simulink library "casper_library_sources"  (Simulink 7.0)
values from neighbouring files (symbols this model uses):
  quant = 'Round  (unbiased: +/- Inf)'    [bus_add_init.m]    (also in bus_addsub_init.m; bus_convert_init.m = 'Round  (unbiased: Even Values)'; bus_maddsub_init.m; bus_mult_init.m)
libraries: xbsIndex_r4 x42, casper_library_sources x2
settings Model: Creator=mdexter  LastModifiedBy=mdexter

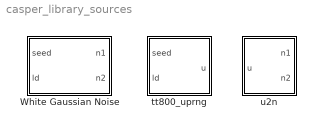
== system casper_library_sources ==
  White Gaussian Noise : Subsystem  mask(White Gaussian Noise Generator){seed=hex2dec('12345678')}
      mask help: Outputs two independent white gaussian noise signals as Fix_17_14 values with standard deviation 1.0, expected value 0.0, and crest factor 3.90625 (125/32).
      mask Help:
      | Initial seed is specified by a mask parameter at design time.  Can be reseeded at runtime by applying a UFix_32_0 value on the seed input and pulsing the load port (ld) high for one cycle.  Holding the load port high for more than one cycle is allowed, but it affects the underlying PRNG in undocumented ways.  Drill down into the subsystem if you want to learn more.
      | 
      | This block uses a TT800 uniform pseudo-random number generator followed by a uniform-to-normal converter implementing the Box-Muller Polar algorithm.
      | 
      | The TT800 is a high quality pseudo-random number generator based on a "twisted generialized linear feedback shift register".  Its output sequence repeats after 2^800 samples (~10^240 samples).  For more info see: Matsumoto, M. and Kurita, Y. 1994. "Twisted GFSR generators II", ACM Trans. Model. Comput. Simul. 4, 3 (Jul. 1994), 254-266 (http://doi.acm.org/10.1145/189443.189445).
      mask CallbackString:
      | if str2num(get_param(gcb, 'seed')) == 0
      |     error('Seed cannot be zero.')
      | end
      mask Display:
      | port_label('input',1,'seed');
      | port_label('input',2,'ld');
      | port_label('output',1,'n1');
      | port_label('output',2,'n2');
  tt800_uprng : Subsystem  mask(TT800 Uniform Psedo-Random Number Generator){seed=hex2dec('12345678')}
      mask help: The TT800 is a high quality pseudo-random number generator based on a "twisted generialized linear feedback shift register". Its output sequence repeats after 2^800 samples (~10^240 samples). For more info see: Matsumoto, M. and Kurita, Y. 1994. "Twisted GFSR generators II", ACM Trans. Model. Comput. Simul. 4, 3 (Jul. 1994), 254-266 (http://doi.acm.org/10.1145/189443.189445).
      mask init:
      | set_param([gcb,'/tt800_seed_gen/LFSR'],'rst_value',sprintf('''%08X''', seed));
      mask Help: Initial seed is specified by a mask parameter at design time.  Can be reseeded at runtime by applying a UFix_32_0 value on the seed input and pulsing the load port (ld) high for one cycle.  Holding the load port high for more than one cycle is allowed, but it affects the generator in undocumented ways.  Drill down into the subsystem if you want to learn more.
      mask Display:
      | port_label('input',1,'seed');
      | port_label('input',2,'ld');
      | port_label('output',1,'u');
  u2n : Subsystem  mask(Uniform to Normal Converter){hideme=off}
      mask prompts: hideme "Hide me"
      mask help: Converts a variable with uniform distribution into two independent normally distributed variables.
      mask Help: Converts a variable with uniform distribution into two independent normally distributed variables.

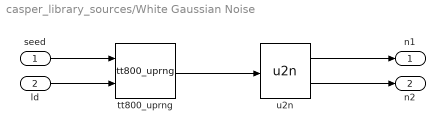
== system casper_library_sources/White Gaussian Noise ==
  seed : Inport  OutDataType=sfix(16)  OutScaling=2^0
  ld : Inport  Port=2  OutDataType=sfix(16)  OutScaling=2^0
  tt800_uprng : casper_library_sources/tt800_uprng  SystemSampleTime=-1  seed=seed
  u2n : casper_library_sources/u2n  SystemSampleTime=-1  hideme=off
  n1 : Outport  OutDataType=sfix(16)  OutScaling=2^0
  n2 : Outport  Port=2  OutDataType=sfix(16)  OutScaling=2^0
  wires:
  tt800_uprng/1 -> u2n/1
  seed/1 -> tt800_uprng/1
  u2n/1 -> n1/1
  ld/1 -> tt800_uprng/2
  u2n/2 -> n2/1

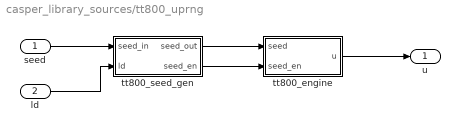
== system casper_library_sources/tt800_uprng ==
  seed : Inport  OutDataType=sfix(16)  OutScaling=2^0
  ld : Inport  Port=2  OutDataType=sfix(16)  OutScaling=2^0
  tt800_engine : Subsystem
  tt800_seed_gen : Subsystem
  u : Outport  OutDataType=sfix(16)  OutScaling=2^0
  wires:
  ld/1 -> tt800_seed_gen/2(ld)
  tt800_engine/1(u) -> u/1
  seed/1 -> tt800_seed_gen/1(seed_in)
  tt800_seed_gen/2(seed_en) -> tt800_engine/2(seed_en)
  tt800_seed_gen/1(seed_out) -> tt800_engine/1(seed)

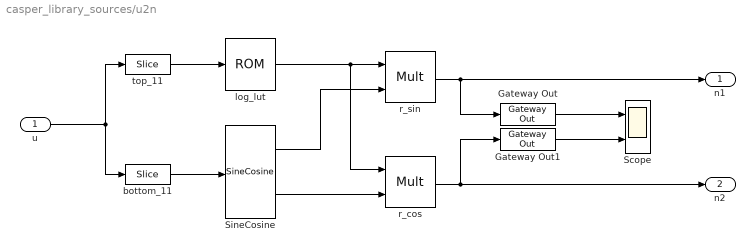
== system casper_library_sources/u2n ==
  u : Inport  OutDataType=sfix(16)  OutScaling=2^0
  Gateway Out : xbsIndex_r4/Gateway Out  hdl_port=off  timing_constraint=None  locs_specified=off  LOCs={}  block_type=gatewayout
      settings: infoedit="Gateway out block.  Converts Xilinx fixed point inputs into ouputs of type Simulink integer, double, or fixed point.<P><P>Hardware notes:  In hardware these blocks become top level output ports or are discarded, depending on how they are configured."  xl_area=[0 0 0 0 17 0 0]  block_version=10.1.3
  Gateway Out1 : xbsIndex_r4/Gateway Out  hdl_port=off  timing_constraint=None  locs_specified=off  LOCs={}  block_type=gatewayout
      settings: infoedit="Gateway out block.  Converts Xilinx fixed point inputs into ouputs of type Simulink integer, double, or fixed point.<P><P>Hardware notes:  In hardware these blocks become top level output ports or are discarded, depending on how they are configured."  xl_area=[0 0 0 0 17 0 0]  block_version=10.1.3
  Scope : Scope  NumInputPorts=2
      settings: YMin=-5~-5  YMax=5~5
  SineCosine : xbsIndex_r4/SineCosine  mode=Sine and Cosine  neg_sin=off  neg_cos=off  n_bits=8  sym_output=off  en=off  latency=2  dbl_ovrd=off  explicit_period=off  period=1  mem_type=Block RAM  pipeline=on  use_rpm=on  block_type=sincos
      settings: xl_area=[8 16 1 2 0 0 0]  block_version=10.1.3
  bottom_11 : xbsIndex_r4/Slice  nbits=11  boolean_output=off  mode=Lower Bit Location + Width  bit1=0  base1=MSB of Input  bit0=0  base0=LSB of Input  dbl_ovrd=off  block_type=slice
      settings: infoedit="Extracts a given range of bits from each input sample and presents it at the output.  The output type is ordinarily unsigned with binary point at zero, but can be Boolean when the slice is one bit wide.<P><P>Hardware notes: In hardware this block costs nothing."  block_version=10.1.3
  log_lut : xbsIndex_r4/ROM  depth=2^11  initVector=quant(sqrt(-2*log(linspace(2^-11,1,2^11))),2^-7)  distributed_mem=Block RAM  rst=off  init_reg=0  en=off  latency=1  arith_type=Unsigned  n_bits=9  bin_pt=7  dbl_ovrd=off  optimize=Area  use_rpm=off  block_type=sprom
      settings: xl_area=[0 0 1 0 0 0 0]  block_version=10.1.3
  r_cos : xbsIndex_r4/Mult  precision=Full  arith_type="Signed  (2's comp)"  n_bits=8  bin_pt=2  quantization=Truncate  overflow=Wrap  en=off  latency=3  dbl_ovrd=off  use_behavioral_HDL=off  use_embedded=on  opt=Speed  optimum_pipeline=off  pipeline=on  use_rpm=on  placement_style=Rectangular shape  block_type=mult
      settings: infoedit=Hardware notes: To use the internal pipeline stage of the dedicated multiplier you must select 'Pipeline for maximum performance'.  xl_area=[18 34 0 17 0 1 0]  block_version=10.1.3
  r_sin : xbsIndex_r4/Mult  precision=Full  arith_type="Signed  (2's comp)"  n_bits=8  bin_pt=2  quantization=Truncate  overflow=Wrap  en=off  latency=3  dbl_ovrd=off  use_behavioral_HDL=off  use_embedded=on  opt=Speed  optimum_pipeline=off  pipeline=on  use_rpm=on  placement_style=Rectangular shape  block_type=mult
      settings: infoedit=Hardware notes: To use the internal pipeline stage of the dedicated multiplier you must select 'Pipeline for maximum performance'.  xl_area=[18 34 0 17 0 1 0]  block_version=10.1.3
  top_11 : xbsIndex_r4/Slice  nbits=11  boolean_output=off  mode=Upper Bit Location + Width  bit1=0  base1=MSB of Input  bit0=0  base0=MSB of Input  dbl_ovrd=off  block_type=slice
      settings: infoedit="Extracts a given range of bits from each input sample and presents it at the output.  The output type is ordinarily unsigned with binary point at zero, but can be Boolean when the slice is one bit wide.<P><P>Hardware notes: In hardware this block costs nothing."  block_version=10.1.3
  n1 : Outport  OutDataType=sfix(16)  OutScaling=2^0
  n2 : Outport  Port=2  OutDataType=sfix(16)  OutScaling=2^0
  wires:
  r_cos/1 -> n2/1, Gateway Out1/1
  r_sin/1 -> n1/1, Gateway Out/1
  SineCosine/1 -> r_sin/2
  log_lut/1 -> r_cos/1, r_sin/1
  SineCosine/2 -> r_cos/2
  u/1 -> bottom_11/1, top_11/1
  top_11/1 -> log_lut/1
  bottom_11/1 -> SineCosine/1
  Gateway Out1/1 -> Scope/2
  Gateway Out/1 -> Scope/1

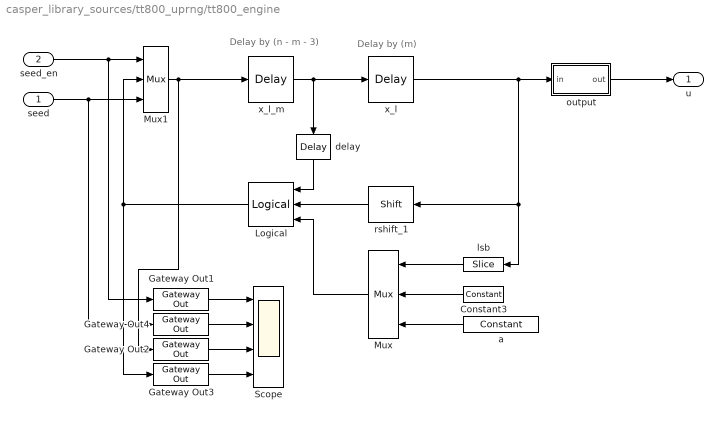
== system casper_library_sources/tt800_uprng/tt800_engine ==
  note: Delay by (m)
  note: Delay by (n - m - 3)
  seed : Inport  OutDataType=sfix(16)  OutScaling=2^0
  seed_en : Inport  Port=2  OutDataType=sfix(16)  OutScaling=2^0
  Constant3 : xbsIndex_r4/Constant  Orientation=left  arith_type=Unsigned  const=0  n_bits=32  bin_pt=0  explicit_period=off  period=1  equ=P=C  opselect=C  inp2=PCIN>>17  opr=+  inp1=P  carry=CIN  dbl_ovrd=off  block_type=constant
  Gateway Out{1..4} (4 alike) : xbsIndex_r4/Gateway Out  hdl_port=off  timing_constraint=None  locs_specified=off  LOCs={}  block_type=gatewayout
      settings: infoedit="Gateway out block.  Converts Xilinx fixed point inputs into ouputs of type Simulink integer, double, or fixed point.<P><P>Hardware notes:  In hardware these blocks become top level output ports or are discarded, depending on how they are configured."  xl_area=[0 0 0 0 0 0 0]  block_version=10.1.3
  Logical : xbsIndex_r4/Logical  Orientation=left  logical_function=XOR  inputs=3  en=off  latency=1  precision=Full  arith_type=Unsigned  n_bits=8  bin_pt=2  align_bp=off  dbl_ovrd=off  block_type=logical
      settings: xl_area=[32 32 0 32 0 0 0]
  Mux : xbsIndex_r4/Mux  Orientation=left  inputs=2  en=off  latency=1  precision=Full  arith_type="Signed  (2's comp)"  n_bits=8  bin_pt=2  quantization=Truncate  overflow=Wrap  dbl_ovrd=off  block_type=mux
      settings: xl_area=[16 32 0 32 0 0 0]
  Mux1 : xbsIndex_r4/Mux  inputs=2  en=off  latency=1  precision=Full  arith_type="Signed  (2's comp)"  n_bits=8  bin_pt=2  quantization=Truncate  overflow=Wrap  dbl_ovrd=off  block_type=mux
      settings: xl_area=[16 32 0 32 0 0 0]
  Scope : Scope  NumInputPorts=4
      settings: YMin=-5~-5~-5~-5  YMax=5~5~5~5
  a : xbsIndex_r4/Constant  Orientation=left  arith_type=Unsigned  const=hex2dec('8EBFD028')  n_bits=32  bin_pt=0  explicit_period=off  period=1  equ=P=C  opselect=C  inp2=PCIN>>17  opr=+  inp1=P  carry=CIN  dbl_ovrd=off  block_type=constant
  delay : xbsIndex_r4/Delay  Orientation=down  en=off  latency=1  dbl_ovrd=off  reg_retiming=off  block_type=delay
      settings: xl_area=[16 32 0 0 0 0 0]
  lsb : xbsIndex_r4/Slice  Orientation=left  nbits=1  boolean_output=off  mode=Lower Bit Location + Width  bit1=0  base1=MSB of Input  bit0=0  base0=LSB of Input  dbl_ovrd=off  block_type=slice
      settings: infoedit="Extracts a given range of bits from each input sample and presents it at the output.  The output type is ordinarily unsigned with binary point at zero, but can be Boolean when the slice is one bit wide.<P><P>Hardware notes: In hardware this block costs nothing."  block_version=10.1.3
  output : Subsystem
  rshift_1 : xbsIndex_r4/Shift  Orientation=left  shift_dir=Right  shift_bits=1  en=off  latency=1  precision=User Defined  arith_type=Unsigned  n_bits=32  bin_pt=0  quantization=Truncate  overflow=Wrap  dbl_ovrd=off  block_type=shift
      settings: xl_area=[0 32 0 0 0 0 0]  block_version=10.1.3
  x_l : xbsIndex_r4/Delay  en=off  latency=7  dbl_ovrd=off  reg_retiming=off  block_type=delay
      settings: xl_area=[16 32 0 32 0 0 0]
  x_l_m : xbsIndex_r4/Delay  en=off  latency=25-7-3  dbl_ovrd=off  reg_retiming=off  block_type=delay
      settings: xl_area=[16 32 0 32 0 0 0]
  u : Outport  OutDataType=sfix(16)  OutScaling=2^0
  wires:
  x_l_m/1 -> x_l/1, delay/1
  x_l/1 -> lsb/1, rshift_1/1, output/1(in)
  lsb/1 -> Mux/1
  Constant3/1 -> Mux/2
  a/1 -> Mux/3
  rshift_1/1 -> Logical/2
  Mux/1 -> Logical/3
  Logical/1 -> Gateway Out3/1, Mux1/2
  Mux1/1 -> x_l_m/1, Gateway Out2/1
  seed_en/1 -> Gateway Out1/1, Mux1/1
  seed/1 -> Gateway Out4/1, Mux1/3
  Gateway Out1/1 -> Scope/1
  Gateway Out4/1 -> Scope/2
  Gateway Out2/1 -> Scope/3
  Gateway Out3/1 -> Scope/4
  output/1(out) -> u/1
  delay/1 -> Logical/1

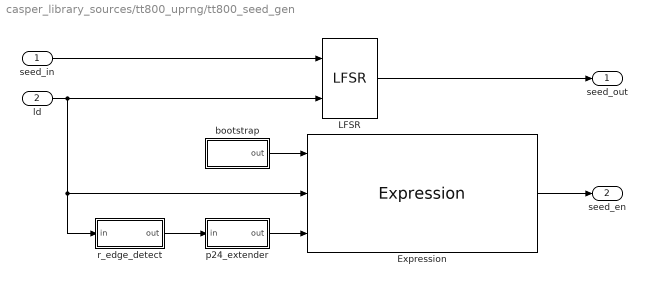
== system casper_library_sources/tt800_uprng/tt800_seed_gen ==
  seed_in : Inport  OutDataType=sfix(16)  OutScaling=2^0
  ld : Inport  Port=2  OutDataType=sfix(16)  OutScaling=2^0
  Expression : xbsIndex_r4/Expression  expression=(bootstrap | ld | ld_ext)  align_bp=on  en=off  latency=1  precision=Full  arith_type=Unsigned  n_bits=8  bin_pt=2  dbl_ovrd=off  block_type=expr
      settings: xl_area=[0, 0, 0, 0, 0, 0, 0]  block_version=10.1.3
  LFSR : xbsIndex_r4/LFSR  lfsr_type=Fibonacci  gate_type=XOR  n_bits=32  polynomial='C0000401'  rst_value='12345678'  rst=off  en=off  reloadable_seed=on  input_type=on  output_type=on  arith_type=Unsigned  bin_pt=0  dbl_ovrd=off  explicit_period=on  period=1  block_type=lfsr
      settings: xl_area=[17 32 0 33 0 0 0]  block_version=10.1.3
  bootstrap : Subsystem
  p24_extender : Subsystem
  r_edge_detect : Subsystem
  seed_out : Outport  OutDataType=sfix(16)  OutScaling=2^0
  seed_en : Outport  Port=2  OutDataType=sfix(16)  OutScaling=2^0
  wires:
  p24_extender/1(out) -> Expression/3
  bootstrap/1(out) -> Expression/1
  LFSR/1 -> seed_out/1
  seed_in/1 -> LFSR/1
  Expression/1 -> seed_en/1
  ld/1 -> Expression/2, r_edge_detect/1(in), LFSR/2
  r_edge_detect/1(out) -> p24_extender/1(in)

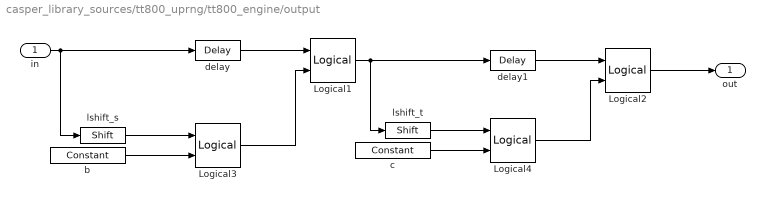
== system casper_library_sources/tt800_uprng/tt800_engine/output ==
  in : Inport  OutDataType=sfix(16)  OutScaling=2^0
  Logical1 : xbsIndex_r4/Logical  logical_function=XOR  inputs=2  en=off  latency=1  precision=Full  arith_type=Unsigned  n_bits=8  bin_pt=2  align_bp=off  dbl_ovrd=off  block_type=logical
      settings: xl_area=[32 32 0 32 0 0 0]
  Logical2 : xbsIndex_r4/Logical  logical_function=XOR  inputs=2  en=off  latency=1  precision=Full  arith_type=Unsigned  n_bits=8  bin_pt=2  align_bp=off  dbl_ovrd=off  block_type=logical
      settings: xl_area=[32 32 0 32 0 0 0]
  Logical3 : xbsIndex_r4/Logical  logical_function=AND  inputs=2  en=off  latency=1  precision=Full  arith_type=Unsigned  n_bits=8  bin_pt=2  align_bp=off  dbl_ovrd=off  block_type=logical
      settings: xl_area=[32 32 0 32 0 0 0]
  Logical4 : xbsIndex_r4/Logical  logical_function=AND  inputs=2  en=off  latency=1  precision=Full  arith_type=Unsigned  n_bits=8  bin_pt=2  align_bp=off  dbl_ovrd=off  block_type=logical
      settings: xl_area=[32 32 0 32 0 0 0]
  b : xbsIndex_r4/Constant  arith_type=Unsigned  const=hex2dec('2B5B2500')  n_bits=32  bin_pt=0  explicit_period=off  period=1  equ=P=C  opselect=C  inp2=PCIN>>17  opr=+  inp1=P  carry=CIN  dbl_ovrd=off  block_type=constant
  c : xbsIndex_r4/Constant  arith_type=Unsigned  const=hex2dec('DB8B0000')  n_bits=32  bin_pt=0  explicit_period=off  period=1  equ=P=C  opselect=C  inp2=PCIN>>17  opr=+  inp1=P  carry=CIN  dbl_ovrd=off  block_type=constant
  delay : xbsIndex_r4/Delay  en=off  latency=1  dbl_ovrd=off  reg_retiming=off  block_type=delay
      settings: xl_area=[16 32 0 0 0 0 0]
  delay1 : xbsIndex_r4/Delay  en=off  latency=1  dbl_ovrd=off  reg_retiming=off  block_type=delay
      settings: xl_area=[16 32 0 0 0 0 0]
  lshift_s : xbsIndex_r4/Shift  shift_dir=Left  shift_bits=7  en=off  latency=0  precision=User Defined  arith_type=Unsigned  n_bits=32  bin_pt=0  quantization=Truncate  overflow=Wrap  dbl_ovrd=off  block_type=shift
      settings: xl_area=[0 0 0 0 0 0 0]  block_version=10.1.3
  lshift_t : xbsIndex_r4/Shift  shift_dir=Left  shift_bits=15  en=off  latency=0  precision=User Defined  arith_type=Unsigned  n_bits=32  bin_pt=0  quantization=Truncate  overflow=Wrap  dbl_ovrd=off  block_type=shift
      settings: xl_area=[0 0 0 0 0 0 0]  block_version=10.1.3
  out : Outport  OutDataType=sfix(16)  OutScaling=2^0
  wires:
  delay/1 -> Logical1/1
  lshift_s/1 -> Logical3/1
  b/1 -> Logical3/2
  Logical3/1 -> Logical1/2
  Logical1/1 -> delay1/1, lshift_t/1
  lshift_t/1 -> Logical4/1
  c/1 -> Logical4/2
  delay1/1 -> Logical2/1
  Logical4/1 -> Logical2/2
  in/1 -> delay/1, lshift_s/1
  Logical2/1 -> out/1

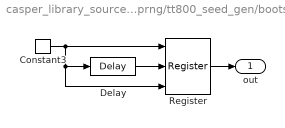
== system casper_library_sources/tt800_uprng/tt800_seed_gen/bootstrap ==
  Constant3 : xbsIndex_r4/Constant  arith_type=Boolean  const=1  n_bits=1  bin_pt=0  explicit_period=on  period=1  equ=P=C  opselect=C  inp2=PCIN>>17  opr=+  inp1=P  carry=CIN  dbl_ovrd=off  block_type=constant
  Delay : xbsIndex_r4/Delay  en=off  latency=25  dbl_ovrd=off  reg_retiming=off  block_type=delay
      settings: xl_area=[2 2 0 2 0 0 0]
  Register : xbsIndex_r4/Register  init=0  rst=on  en=on  dbl_ovrd=off  block_type=register
      settings: xl_area=[1 1 0 0 0 0 0]
  out : Outport  OutDataType=sfix(16)  OutScaling=2^0
  wires:
  Register/1 -> out/1
  Constant3/1 -> Register/3, Delay/1, Register/1
  Delay/1 -> Register/2

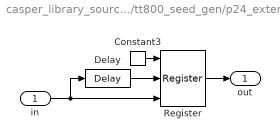
== system casper_library_sources/tt800_uprng/tt800_seed_gen/p24_extender ==
  in : Inport  OutDataType=sfix(16)  OutScaling=2^0
  Constant3 : xbsIndex_r4/Constant  arith_type=Boolean  const=1  n_bits=1  bin_pt=0  explicit_period=on  period=1  equ=P=C  opselect=C  inp2=PCIN>>17  opr=+  inp1=P  carry=CIN  dbl_ovrd=off  block_type=constant
  Delay : xbsIndex_r4/Delay  en=off  latency=24  dbl_ovrd=off  reg_retiming=off  block_type=delay
      settings: xl_area=[2 2 0 2 0 0 0]
  Register : xbsIndex_r4/Register  init=0  rst=on  en=on  dbl_ovrd=off  block_type=register
      settings: xl_area=[1 1 0 0 0 0 0]
  out : Outport  OutDataType=sfix(16)  OutScaling=2^0
  wires:
  Register/1 -> out/1
  Constant3/1 -> Register/1
  Delay/1 -> Register/2
  in/1 -> Register/3, Delay/1

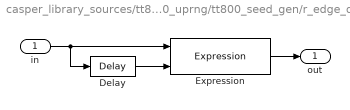
== system casper_library_sources/tt800_uprng/tt800_seed_gen/r_edge_detect ==
  in : Inport  OutDataType=sfix(16)  OutScaling=2^0
  Delay : xbsIndex_r4/Delay  en=off  latency=1  dbl_ovrd=off  reg_retiming=off  block_type=delay
  Expression : xbsIndex_r4/Expression  expression=curr & ~prev  align_bp=on  en=off  latency=0  precision=Full  arith_type=Unsigned  n_bits=16  bin_pt=0  dbl_ovrd=off  block_type=expr
      settings: block_version=10.1.3
  out : Outport  OutDataType=sfix(16)  OutScaling=2^0
  wires:
  Expression/1 -> out/1
  Delay/1 -> Expression/2
  in/1 -> Expression/1, Delay/1
